simulink model "Rot_to_Euler"  (R2018b)
settings: Solver=VariableStepAuto  StartTime=0.0  StopTime=10.0  RelTol=1e-3
libraries: robotcorelib x2
settings Model: Creator=woo  LastModifiedBy=im-lab

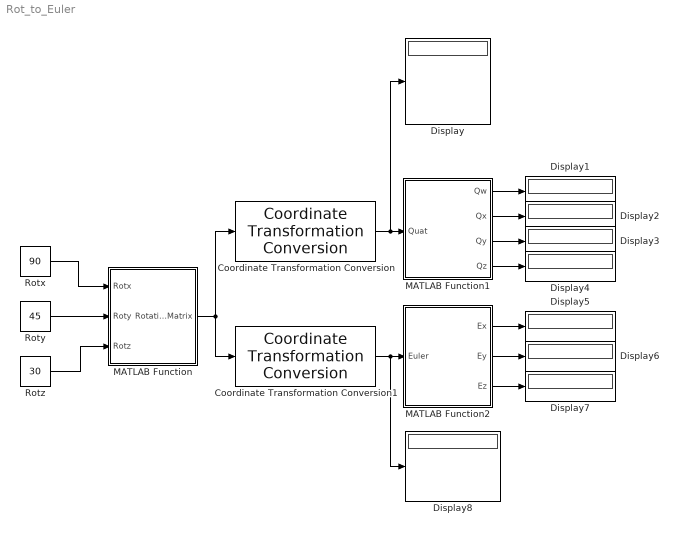
== system Rot_to_Euler ==
  Coordinate Transformation Conversion : robotcorelib/Coordinate Transformation Conversion  InputRepresentation=Rotation Matrix  InputEulerSequence=ZYX  ShowTrVecInputPort=on  OutputRepresentation=Quaternion  OutputEulerSequence=ZYX  ShowTrVecOutputPort=on  SimulateUsing=Interpreted execution
      settings: SourceProductBaseCode=RO
  Coordinate Transformation Conversion1 : robotcorelib/Coordinate Transformation Conversion  InputRepresentation=Rotation Matrix  InputEulerSequence=ZYX  ShowTrVecInputPort=on  OutputRepresentation=Euler Angles  OutputEulerSequence=XYZ  ShowTrVecOutputPort=on  SimulateUsing=Interpreted execution
      settings: SourceProductBaseCode=RO
  Display{,1..8} (9 alike) : Display
  MATLAB Function : MATLAB Function  TreatAsAtomicUnit=on
  MATLAB Function1 : MATLAB Function  TreatAsAtomicUnit=on
  MATLAB Function2 : MATLAB Function  TreatAsAtomicUnit=on
  Rotx : Constant  Value=90
  Roty : Constant  Value=45
  Rotz : Constant  Value=30
  wires:
  Rotx/1 -> MATLAB Function/1(Rotx)
  Roty/1 -> MATLAB Function/2(Roty)
  Rotz/1 -> MATLAB Function/3(Rotz)
  MATLAB Function/1(RotationMatrix) -> Coordinate Transformation Conversion/1, Coordinate Transformation Conversion1/1
  Coordinate Transformation Conversion/1 -> Display/1, MATLAB Function1/1(Quat)
  Coordinate Transformation Conversion1/1 -> Display8/1, MATLAB Function2/1(Euler)
  MATLAB Function1/1(Qw) -> Display1/1
  MATLAB Function1/2(Qx) -> Display2/1
  MATLAB Function1/3(Qy) -> Display3/1
  MATLAB Function1/4(Qz) -> Display4/1
  MATLAB Function2/1(Ex) -> Display5/1
  MATLAB Function2/2(Ey) -> Display6/1
  MATLAB Function2/3(Ez) -> Display7/1

== matlab function Rot_to_Euler/MATLAB Function1 ==
  data: Quat input; Qw output; Qx output; Qy output; Qz output
function [Qw,Qx,Qy,Qz]= fcn(Quat)

Qw = Quat(1,1);
Qx = Quat(2,1);
Qy = Quat(3,1);
Qz = Quat(4,1);

== matlab function Rot_to_Euler/MATLAB Function ==
  data: Rotx input; RotationMatrix output; Roty input; Rotz input
function RotationMatrix = fcn(Rotx,Roty,Rotz)

Rx = [1,0,0; 0,cos(Rotx),-sin(Rotx); 0,sin(Rotx),cos(Rotx);];
Ry = [cos(Roty),0,sin(Roty); 0,1,0; -sin(Roty),0,cos(Roty);];
Rz = [cos(Rotz),-sin(Rotz),0; sin(Rotz),cos(Rotz),0; 0,0,1;];



RotationMatrix = Rx*Ry*Rz;

== matlab function Rot_to_Euler/MATLAB Function2 ==
  data: Euler input; Ex output; Ey output; Ez output
function [Ex,Ey,Ez]= fcn(Euler)

Ex = Euler(1,1);
Ey = Euler(2,1);
Ez = Euler(3,1);
